simulink model "IEEE_39bus_genout"  (R2021a)
settings: Solver=ode3  StartTime=0.0  StopTime=100  FixedStep=Ts  MaxStep=1/60  RelTol=1e-2  AbsTol=1e-1
PreLoadFcn:
  | Ts=50e-6; ssn_ieee39_params; dec=20;
InitFcn:
  | Ts=50e-6; ssn_ieee39_params; dec=20;
values from neighbouring files (symbols this model uses):
  f = 50    [ssn_ieee39_params_ctrl.m]
  fNom = f    (= 60)    [ssn_ieee39_params_ctrl.m]
  ILR = 5.02    [ssn_ieee39_params_ctrl.m]
  IQMIN = 0.1    [ssn_ieee39_params_ctrl.m]
  ISCLIM = 1    [ssn_ieee39_params_ctrl.m]
  ITFpu = 1.10    (= 1.1)    [ssn_ieee39_params_ctrl.m]
  K = 1    [ssn_ieee39_params_ctrl.m]
  K1 = 1    [ssn_ieee39_params_ctrl.m]
  K2 = 2    [ssn_ieee39_params_ctrl.m]
  KCL = 1.04    [ssn_ieee39_params_ctrl.m]
  KFB = 0    [ssn_ieee39_params_ctrl.m]
  KFF = 1    [ssn_ieee39_params_ctrl.m]
  KFIX = 1    [ssn_ieee39_params_ctrl.m]
  KG = 1    [ssn_ieee39_params_ctrl.m]
  KIA = 59.91    [ssn_ieee39_params_ctrl.m]
  KIOEX = 0.0303    [ssn_ieee39_params_ctrl.m]
  KIUEX = 0.0303    [ssn_ieee39_params_ctrl.m]
  KIUOEX = 1    [ssn_ieee39_params_ctrl.m]
  KIUUEX = 1    [ssn_ieee39_params_ctrl.m]
  KLR = 22.47    [ssn_ieee39_params_ctrl.m]
  KM = 1    [ssn_ieee39_params_ctrl.m]
  KOEL = 0.24    [ssn_ieee39_params_ctrl.m]
  Kp = 1    [ssn_ieee39_params_ctrl.m]
  KPA = 30    [ssn_ieee39_params_ctrl.m]
  KPOEL = 1    [ssn_ieee39_params_ctrl.m]
  KPOEX = 0    [ssn_ieee39_params_ctrl.m]
  KPUEX = 0    [ssn_ieee39_params_ctrl.m]
  KSCALE = 0.319    [ssn_ieee39_params_ctrl.m]
  KUF = 0    [ssn_ieee39_params_ctrl.m]
  KUI = 0.001    [ssn_ieee39_params_ctrl.m]
  KUL = 0.24    [ssn_ieee39_params_ctrl.m]
  s = 10    [ssn_ieee39_params_ctrl.m]
  TA = 0.01    [ssn_ieee39_params_ctrl.m]
  Tadj = 0    [ssn_ieee39_params_ctrl.m]
  taps = [1 1 1.07 1.07 1.009 1.025 1 1.025 1.025 1.025]*1    [ssn_ieee39_params_ctrl.m]
  TF = 0.02    [ssn_ieee39_params_ctrl.m]
  TG = 0.024    [ssn_ieee39_params_ctrl.m]
  TINV = 0    [ssn_ieee39_params_ctrl.m]
  TIT = 0.1    [ssn_ieee39_params_ctrl.m]
  TL_10_11_len = 14    [ssn_ieee39_params_ctrl.m]
  TL_10_13_len = 14    [ssn_ieee39_params_ctrl.m]
  TL_13_14_len = 32    [ssn_ieee39_params_ctrl.m]
  TL_14_15_len = 70    [ssn_ieee39_params_ctrl.m]
  TL_15_16_len = 31.5    [ssn_ieee39_params_ctrl.m]
  TL_16_17_len = 26    [ssn_ieee39_params_ctrl.m]
  TL_16_19_len = 61    [ssn_ieee39_params_ctrl.m]
  TL_16_21_len = 46    [ssn_ieee39_params_ctrl.m]
  TL_16_24_len = 15    [ssn_ieee39_params_ctrl.m]
  TL_17_18_len = 26    [ssn_ieee39_params_ctrl.m]
  TL_17_27_len = 59    [ssn_ieee39_params_ctrl.m]
  TL_1_2_len = 134    [ssn_ieee39_params_ctrl.m]
  TL_1_39_len = 105    [ssn_ieee39_params_ctrl.m]
  TL_21_22_len = 47    [ssn_ieee39_params_ctrl.m]
  TL_22_23_len = 33    [ssn_ieee39_params_ctrl.m]
  TL_24_23_len = 88    [ssn_ieee39_params_ctrl.m]
  TL_25_26_len = 101    [ssn_ieee39_params_ctrl.m]
  TL_26_27_len = 46.5    [ssn_ieee39_params_ctrl.m]
  TL_26_28_len = 151    [ssn_ieee39_params_ctrl.m]
  TL_26_29_len = 200    [ssn_ieee39_params_ctrl.m]
  TL_28_29_len = 48    [ssn_ieee39_params_ctrl.m]
  TL_2_25_len = 28    [ssn_ieee39_params_ctrl.m]
  TL_2_2_len = 49    [ssn_ieee39_params_ctrl.m]
  TL_3_18_len = 42    [ssn_ieee39_params_ctrl.m]
  TL_3_4_len = 53    [ssn_ieee39_params_ctrl.m]
  TL_4_14_len = 33    [ssn_ieee39_params_ctrl.m]
  TL_4_5_len = 32.5    [ssn_ieee39_params_ctrl.m]
  TL_5_6_len = 14    [ssn_ieee39_params_ctrl.m]
  TL_5_8_len = 32    [ssn_ieee39_params_ctrl.m]
  TL_6_11_len = 26.5    [ssn_ieee39_params_ctrl.m]
  TL_6_7_len = 25.5    [ssn_ieee39_params_ctrl.m]
  TL_7_8_len = 15    [ssn_ieee39_params_ctrl.m]
  TL_8_9_len = 93    [ssn_ieee39_params_ctrl.m]
  TL_9_39_len = 136    [ssn_ieee39_params_ctrl.m]
  TOEL = 5.00    (= 5)    [ssn_ieee39_params_ctrl.m]
  TQREF = 0    [ssn_ieee39_params_ctrl.m]
  TQSCL = 0.012    [ssn_ieee39_params_ctrl.m]
  Ts_PMU = 1/1000    (= 0.001)    [ssn_ieee39_params_ctrl.m]
  TU1 = 0    [ssn_ieee39_params_ctrl.m]
  TU2 = 0    [ssn_ieee39_params_ctrl.m]
  TU3 = 0    [ssn_ieee39_params_ctrl.m]
  TU4 = 0    [ssn_ieee39_params_ctrl.m]
  TUL = 0    [ssn_ieee39_params_ctrl.m]
  TUP = 0.050    (= 0.05)    [ssn_ieee39_params_ctrl.m]
  TUQ = .005    (= 0.005)    [ssn_ieee39_params_ctrl.m]
  TUV = 0.2    [ssn_ieee39_params_ctrl.m]
  VAAMAX = VAMAX    (= 7.05)    [ssn_ieee39_params_ctrl.m]
  VAMAX = 7.05    [ssn_ieee39_params_ctrl.m]
  VAMIN = -6.11    [ssn_ieee39_params_ctrl.m]
  VBMAX = 999    [ssn_ieee39_params_ctrl.m]
  VF = 0    [ssn_ieee39_params_ctrl.m]
  VFB = 0    [ssn_ieee39_params_ctrl.m]
  VMMAX = 7.05    [ssn_ieee39_params_ctrl.m]
  VMMIN = -6.11    [ssn_ieee39_params_ctrl.m]
  VOELmax1 = 0.2353    [ssn_ieee39_params_ctrl.m]
  VOELmax2 = 0.0    (= 0)    [ssn_ieee39_params_ctrl.m]
  VOELmin1 = -0.24    [ssn_ieee39_params_ctrl.m]
  VOELmin2 = -1.0    (= -1)    [ssn_ieee39_params_ctrl.m]
  VRMAX = 7.05    [ssn_ieee39_params_ctrl.m]
  VRMIN = -6.11    [ssn_ieee39_params_ctrl.m]
  VSCLmax = 0.20    (= 0.2)    [ssn_ieee39_params_ctrl.m]
  VSCLmin = -0.10    (= -0.1)    [ssn_ieee39_params_ctrl.m]
  VUELmax1 = 1    [ssn_ieee39_params_ctrl.m]
  VUELmax2 = 1    [ssn_ieee39_params_ctrl.m]
  VUELmin1 = -1    [ssn_ieee39_params_ctrl.m]
  VUELmin2 = -1    [ssn_ieee39_params_ctrl.m]
  VUImax = 1    [ssn_ieee39_params_ctrl.m]
  VUImin = -1    [ssn_ieee39_params_ctrl.m]
undefined symbols (not defined in the file or in its folder): D1, Delta, MOV_segment9, powergui
libraries: spsThreePhaseVIMeasurementLib x42, slpidlib x40, powerlib_extras x30, op_dpl_lib x30, simulink_extras x20, spsST2AModel x20, spsThreePhaseParallelRLCLoadLib x19, spsThreePhaseTransformerTwoWindingsLib x13, spsSynchronousMachinepuStandardLib x10, simulink x10, spsPower3phInstantaneousLib x10, spsThreePhasePISectionLineLib x7
(part 5 of 12)

== system IEEE_39bus_genout/SM_master/G6/G6 ==
  note: Rotor Speed
  note: Rotor Speed Reference
  note: SM Measurement Signal
  note: Active Power
  note: Field Current
  note: Voltage Reference
  note: Stator Voltage
  note: Reactive Power
  note: Stator Current
  note: Field Voltage (Vf)
  note: Mechanical
      | Power (Pm)
  note: Measurement Outputs
  note: Rotor Speed
  note: Active Power
  note: Stator Voltage
  note: Stator Current
  note: Field Current
  note: Reactive Power
  wref (pu) : Inport
  Vref (pu) : Inport  Port=2
  Generator Measurements (Output) : Subsystem
  Governor model with Droop : Subsystem
  Ground7 : Ground
  ST6C EXCITER-1 : Subsystem
  Synchronous Machine : spsSynchronousMachinepuStandardLib/Synchronous Machine pu Standard  PresetModel=No  MechanicalLoad=Mechanical power Pm  ShowDetailedParameters=on  RotorType=Salient-pole  Units=per unit standard parameters  MeasurementBus=off  NominalParameters="[ Pn  Vn   f ]"  Reactances1=[ 31 32 33 34 35 36 37 ]  Reactances2=[ 1.305, 0.296, 0.252, 0.474, 0.243, 0.18 ]  dAxisTimeConstants=Short-circuit  qAxisTimeConstants=Open-circuit  TimeConstants1=[]  TimeConstants2=[]  TimeConstants3=[]  TimeConstants4=[]  TimeConstants5=[ 1.01, 0.053, 0.1 ]  TimeConstants6=[]  TimeConstants7=[]  TimeConstants8=[]  StatorResistance=2.8544e-3  Mechanical=[H1 0 2]  PolePairs=2  InitialConditions=[0 -62.5202 1.01055 1.01055 1.01055 8.25986 -111.74 128.26 1.32748]  SetSaturation=off  Saturation=[0.6404,0.7127,0.8441,0.9214,0.9956,1.082,1.19,1.316,1.457;0.7,0.7698,0.8872,0.9466,0.9969,1.046,1.1,1.151,1.201]  LoadFlowParameters=[1 150000000 0 0]  TsPowergui=0  TsBlock=-1  IterativeModel=Trapezoidal non iterative  IterativeDiscreteModel=Trapezoidal non iterative  BusType=PV  Pref=42e6  Qref=0  Qmin=-50000000  Qmax=50000000  PLF=0  QLF=0
      settings: SourceProductBaseCode=PS
  A : PMIOPort  Side=Right
  B : PMIOPort  Port=2  Side=Right
  C : PMIOPort  Port=3  Side=Right
  sm1 : Outport  VectorParamsAs1DForOutWhenUnconnected=off
  wires:
  [PT1st] -> Governor model with Droop/3(Input)
  [Ifd1st] -> ST6C EXCITER-1/4(Ifd)
  [Vt1st] -> ST6C EXCITER-1/2(Vt)
  [wm1] -> Governor model with Droop/2(w (pu))
  Generator Measurements (Output)/3(Vt) -> [Vt1st]
  Generator Measurements (Output)/6(PT) -> [PT1st]
  Generator Measurements (Output)/7(QT) -> [QT1st]
  Generator Measurements (Output)/1(sm) -> sm1/1
  Generator Measurements (Output)/5(It) -> [It1st]
  Generator Measurements (Output)/4(Ifd) -> [Ifd1st]
  Generator Measurements (Output)/2(wm) -> [wm1]
  ST6C EXCITER-1/1(Efd) -> Synchronous Machine/2, [Efd1st]
  [PT1st] -> ST6C EXCITER-1/7(PT)
  [It1st] -> ST6C EXCITER-1/3(It)
  [QT1st] -> ST6C EXCITER-1/6(QT)
  Ground7/1 -> ST6C EXCITER-1/5(Vstab)
  wref (pu)/1 -> Governor model with Droop/1(wref (pu)1)
  Governor model with Droop/1(Pmec (pu)) -> Synchronous Machine/1
  Vref (pu)/1 -> ST6C EXCITER-1/1(Vref)
  Synchronous Machine/1 -> Generator Measurements (Output)/1(m)
  connections:
  A/RConn1 -- Synchronous Machine/RConn1
  C/RConn1 -- Synchronous Machine/RConn3
  B/RConn1 -- Synchronous Machine/RConn2

== system IEEE_39bus_genout/SM_master/G7/G7 ==
  note: Rotor Speed
  note: Rotor Speed Reference
  note: SM Measurement Signal
  note: Active Power
  note: Field Current
  note: Voltage Reference
  note: Stator Voltage
  note: Reactive Power
  note: Stator Current
  note: Field Voltage (Vf)
  note: Mechanical
      | Power (Pm)
  note: Measurement Outputs
  note: Rotor Speed
  note: Active Power
  note: Stator Voltage
  note: Stator Current
  note: Field Current
  note: Reactive Power
  wref (pu) : Inport
  Vref (pu) : Inport  Port=2
  Generator Measurements (Output) : Subsystem
  Governor model with Droop : Subsystem
  Ground7 : Ground
  ST6C EXCITER-1 : Subsystem
  Synchronous Machine : spsSynchronousMachinepuStandardLib/Synchronous Machine pu Standard  PresetModel=No  MechanicalLoad=Mechanical power Pm  ShowDetailedParameters=on  RotorType=Salient-pole  Units=per unit standard parameters  MeasurementBus=off  NominalParameters="[ Pn  Vn   f ]"  Reactances1=[ 31 32 33 34 35 36 37 ]  Reactances2=[ 1.305, 0.296, 0.252, 0.474, 0.243, 0.18 ]  dAxisTimeConstants=Short-circuit  qAxisTimeConstants=Open-circuit  TimeConstants1=[]  TimeConstants2=[]  TimeConstants3=[]  TimeConstants4=[]  TimeConstants5=[ 1.01, 0.053, 0.1 ]  TimeConstants6=[]  TimeConstants7=[]  TimeConstants8=[]  StatorResistance=2.8544e-3  Mechanical=[H1 0 2]  PolePairs=2  InitialConditions=[0 -62.5202 1.01055 1.01055 1.01055 8.25986 -111.74 128.26 1.32748]  SetSaturation=off  Saturation=[0.6404,0.7127,0.8441,0.9214,0.9956,1.082,1.19,1.316,1.457;0.7,0.7698,0.8872,0.9466,0.9969,1.046,1.1,1.151,1.201]  LoadFlowParameters=[1 150000000 0 0]  TsPowergui=0  TsBlock=-1  IterativeModel=Trapezoidal non iterative  IterativeDiscreteModel=Trapezoidal non iterative  BusType=PV  Pref=42e6  Qref=0  Qmin=-50000000  Qmax=50000000  PLF=0  QLF=0
      settings: SourceProductBaseCode=PS
  A : PMIOPort  Side=Right
  B : PMIOPort  Port=2  Side=Right
  C : PMIOPort  Port=3  Side=Right
  sm1 : Outport  VectorParamsAs1DForOutWhenUnconnected=off
  wires:
  [PT1st] -> Governor model with Droop/3(Input)
  [Ifd1st] -> ST6C EXCITER-1/4(Ifd)
  [Vt1st] -> ST6C EXCITER-1/2(Vt)
  [wm1] -> Governor model with Droop/2(w (pu))
  Generator Measurements (Output)/3(Vt) -> [Vt1st]
  Generator Measurements (Output)/6(PT) -> [PT1st]
  Generator Measurements (Output)/7(QT) -> [QT1st]
  Generator Measurements (Output)/1(sm) -> sm1/1
  Generator Measurements (Output)/5(It) -> [It1st]
  Generator Measurements (Output)/4(Ifd) -> [Ifd1st]
  Generator Measurements (Output)/2(wm) -> [wm1]
  ST6C EXCITER-1/1(Efd) -> Synchronous Machine/2, [Efd1st]
  [PT1st] -> ST6C EXCITER-1/7(PT)
  [It1st] -> ST6C EXCITER-1/3(It)
  [QT1st] -> ST6C EXCITER-1/6(QT)
  Ground7/1 -> ST6C EXCITER-1/5(Vstab)
  wref (pu)/1 -> Governor model with Droop/1(wref (pu)1)
  Governor model with Droop/1(Pmec (pu)) -> Synchronous Machine/1
  Vref (pu)/1 -> ST6C EXCITER-1/1(Vref)
  Synchronous Machine/1 -> Generator Measurements (Output)/1(m)
  connections:
  A/RConn1 -- Synchronous Machine/RConn1
  C/RConn1 -- Synchronous Machine/RConn3
  B/RConn1 -- Synchronous Machine/RConn2

== system IEEE_39bus_genout/SM_master/G8/ G8 ==
  note: Reactive Power
  note: Field Current
  note: Stator Current
  note: Stator Voltage
  note: Active Power
  note: Rotor Speed
  note: Measurement Outputs
  note: Mechanical
      | Power (PU)
  note: Field Voltage (Vf PU)
  note: Stator Current
  note: Reactive Power
  note: Stator Voltage
  note: Voltage Reference
  note: Field Current
  note: Active Power
  note: SM Measurement Signal
  note: Rotor Speed Reference
  note: Rotor Speed
  wref (pu) : Inport
  Vref (pu) : Inport  Port=2
  "Generator Measurements " : Subsystem
  "Governor model " : Subsystem
  Ground7 : Ground
  ST6C EXCITER-1 : Subsystem
  Synchronous Machine : spsSynchronousMachinepuStandardLib/Synchronous Machine pu Standard  PresetModel=No  MechanicalLoad=Mechanical power Pm  ShowDetailedParameters=on  RotorType=Salient-pole  Units=per unit standard parameters  MeasurementBus=off  NominalParameters="[ Pn  Vn   f ]"  Reactances1=[ 31 32 33 34 35 36 37 ]  Reactances2=[ 1.305, 0.296, 0.252, 0.474, 0.243, 0.18 ]  dAxisTimeConstants=Short-circuit  qAxisTimeConstants=Open-circuit  TimeConstants1=[]  TimeConstants2=[]  TimeConstants3=[]  TimeConstants4=[]  TimeConstants5=[ 1.01, 0.053, 0.1 ]  TimeConstants6=[]  TimeConstants7=[]  TimeConstants8=[]  StatorResistance=2.8544e-3  Mechanical=[H1 0 2]  PolePairs=2  InitialConditions=[0 -62.5202 1.01055 1.01055 1.01055 8.25986 -111.74 128.26 1.32748]  SetSaturation=off  Saturation=[0.6404,0.7127,0.8441,0.9214,0.9956,1.082,1.19,1.316,1.457;0.7,0.7698,0.8872,0.9466,0.9969,1.046,1.1,1.151,1.201]  LoadFlowParameters=[1 150000000 0 0]  TsPowergui=0  TsBlock=-1  IterativeModel=Trapezoidal non iterative  IterativeDiscreteModel=Trapezoidal non iterative  BusType=PV  Pref=42e6  Qref=0  Qmin=-50000000  Qmax=50000000  PLF=0  QLF=0
      settings: SourceProductBaseCode=PS
  A : PMIOPort  Side=Right
  B : PMIOPort  Port=2  Side=Right
  C : PMIOPort  Port=3  Side=Right
  sm1 : Outport  VectorParamsAs1DForOutWhenUnconnected=off
  wires:
  Synchronous Machine/1 -> "Generator Measurements "/1(m)
  Vref (pu)/1 -> ST6C EXCITER-1/1(Vref)
  "Governor model "/1(Pmec (pu)) -> Synchronous Machine/1
  wref (pu)/1 -> "Governor model "/1(wref (pu)1)
  Ground7/1 -> ST6C EXCITER-1/5(Vstab)
  [QT1st] -> ST6C EXCITER-1/6(QT)
  [It1st] -> ST6C EXCITER-1/3(It)
  [PT1st] -> ST6C EXCITER-1/7(PT)
  ST6C EXCITER-1/1(Efd) -> [Efd1st], Synchronous Machine/2
  "Generator Measurements "/2(wm) -> [wm1]
  "Generator Measurements "/4(Ifd) -> [Ifd1st]
  "Generator Measurements "/5(It) -> [It1st]
  "Generator Measurements "/1(sm) -> sm1/1
  "Generator Measurements "/7(QT) -> [QT1st]
  "Generator Measurements "/6(PT) -> [PT1st]
  "Generator Measurements "/3(Vt) -> [Vt1st]
  [wm1] -> "Governor model "/2(w (pu))
  [Vt1st] -> ST6C EXCITER-1/2(Vt)
  [Ifd1st] -> ST6C EXCITER-1/4(Ifd)
  [PT1st] -> "Governor model "/3(Input)
  connections:
  B/RConn1 -- Synchronous Machine/RConn2
  C/RConn1 -- Synchronous Machine/RConn3
  A/RConn1 -- Synchronous Machine/RConn1

== system IEEE_39bus_genout/SM_master/G9/G9 ==
  note: Rotor Speed
  note: Rotor Speed Reference
  note: SM Measurement Signal
  note: Active Power
  note: Field Current
  note: Voltage Reference
  note: Stator Voltage
  note: Reactive Power
  note: Stator Current
  note: Field Voltage (Vf)
  note: Mechanical
      | Power (Pm)
  note: Measurement Outputs
  note: Rotor Speed
  note: Active Power
  note: Stator Voltage
  note: Stator Current
  note: Field Current
  note: Reactive Power
  wref (pu) : Inport
  Vref (pu) : Inport  Port=2
  Generator Measurements (Output) : Subsystem
  Governor model with Droop : Subsystem
  Ground7 : Ground
  ST6C EXCITER-1 : Subsystem
  Synchronous Machine : spsSynchronousMachinepuStandardLib/Synchronous Machine pu Standard  PresetModel=No  MechanicalLoad=Mechanical power Pm  ShowDetailedParameters=on  RotorType=Salient-pole  Units=per unit standard parameters  MeasurementBus=off  NominalParameters="[ Pn  Vn   f ]"  Reactances1=[ 31 32 33 34 35 36 37 ]  Reactances2=[ 1.305, 0.296, 0.252, 0.474, 0.243, 0.18 ]  dAxisTimeConstants=Short-circuit  qAxisTimeConstants=Open-circuit  TimeConstants1=[]  TimeConstants2=[]  TimeConstants3=[]  TimeConstants4=[]  TimeConstants5=[ 1.01, 0.053, 0.1 ]  TimeConstants6=[]  TimeConstants7=[]  TimeConstants8=[]  StatorResistance=2.8544e-3  Mechanical=[H1 0 2]  PolePairs=2  InitialConditions=[0 -62.5202 1.01055 1.01055 1.01055 8.25986 -111.74 128.26 1.32748]  SetSaturation=off  Saturation=[0.6404,0.7127,0.8441,0.9214,0.9956,1.082,1.19,1.316,1.457;0.7,0.7698,0.8872,0.9466,0.9969,1.046,1.1,1.151,1.201]  LoadFlowParameters=[1 150000000 0 0]  TsPowergui=0  TsBlock=-1  IterativeModel=Trapezoidal non iterative  IterativeDiscreteModel=Trapezoidal non iterative  BusType=PV  Pref=42e6  Qref=0  Qmin=-50000000  Qmax=50000000  PLF=0  QLF=0
      settings: SourceProductBaseCode=PS
  A : PMIOPort  Side=Right
  B : PMIOPort  Port=2  Side=Right
  C : PMIOPort  Port=3  Side=Right
  sm1 : Outport  VectorParamsAs1DForOutWhenUnconnected=off
  wires:
  [PT1st] -> Governor model with Droop/3(Input)
  [Ifd1st] -> ST6C EXCITER-1/4(Ifd)
  [Vt1st] -> ST6C EXCITER-1/2(Vt)
  [wm1] -> Governor model with Droop/2(w (pu))
  Generator Measurements (Output)/3(Vt) -> [Vt1st]
  Generator Measurements (Output)/6(PT) -> [PT1st]
  Generator Measurements (Output)/7(QT) -> [QT1st]
  Generator Measurements (Output)/1(sm) -> sm1/1
  Generator Measurements (Output)/5(It) -> [It1st]
  Generator Measurements (Output)/4(Ifd) -> [Ifd1st]
  Generator Measurements (Output)/2(wm) -> [wm1]
  ST6C EXCITER-1/1(Efd) -> Synchronous Machine/2, [Efd1st]
  [PT1st] -> ST6C EXCITER-1/7(PT)
  [It1st] -> ST6C EXCITER-1/3(It)
  [QT1st] -> ST6C EXCITER-1/6(QT)
  Ground7/1 -> ST6C EXCITER-1/5(Vstab)
  wref (pu)/1 -> Governor model with Droop/1(wref (pu)1)
  Governor model with Droop/1(Pmec (pu)) -> Synchronous Machine/1
  Vref (pu)/1 -> ST6C EXCITER-1/1(Vref)
  Synchronous Machine/1 -> Generator Measurements (Output)/1(m)
  connections:
  A/RConn1 -- Synchronous Machine/RConn1
  C/RConn1 -- Synchronous Machine/RConn3
  B/RConn1 -- Synchronous Machine/RConn2

== system IEEE_39bus_genout/powergui/EquivalentModel1/Sources ==
  Mux : Mux  Inputs=[1 1 1 1 1 1 1 1 1]
  u : Outport  VectorParamsAs1DForOutWhenUnconnected=off
  wires:
  Mux/1 -> u/1
  [T82_6949_9359448767590] -> Mux/1
  [T82_6950_9360569412504] -> Mux/2
  [T82_6951_9361932985223] -> Mux/3
  [T82_6951_9356282672159] -> Mux/4
  [T82_6952_9357399545649] -> Mux/5
  [T82_6953_9358759346944] -> Mux/6
  [T82_6951_9355573673919] -> Mux/7
  [T82_6952_9356690586475] -> Mux/8
  [T82_6953_9358050426837] -> Mux/9

== system IEEE_39bus_genout/powergui/EquivalentModel1/Yout ==
  v,i : Inport
  Demux : Demux  Outputs=[1 1 1 1 1 1 1 1 1 1 1 1]
  tag scope: T62_5432_5647820575465=global, T62_5433_5649868956552=global, T62_5434_5652472850936=global, T85_7307_11114326970370=global, T85_7308_11114868792739=global, T85_7309_11109720818426=global, T85_7309_11110395395566=global, T85_7309_11115651114168=global, T85_7310_11110259123535=global, T85_7310_11110933663860=global, T85_7311_11111037927703=global, T85_7311_11111712431213=global
  wires:
  v,i/1 -> Demux/1
  Demux/1 -> [T62_5432_5647820575465]
  Demux/2 -> [T62_5434_5652472850936]
  Demux/3 -> [T62_5433_5649868956552]
  Demux/4 -> [T85_7307_11114326970370]
  Demux/5 -> [T85_7308_11114868792739]
  Demux/6 -> [T85_7309_11115651114168]
  Demux/7 -> [T85_7309_11110395395566]
  Demux/8 -> [T85_7310_11110933663860]
  Demux/9 -> [T85_7311_11111712431213]
  Demux/10 -> [T85_7309_11109720818426]
  Demux/11 -> [T85_7310_11110259123535]
  Demux/12 -> [T85_7311_11111037927703]

== system IEEE_39bus_genout/powergui/EquivalentModel10/Sources ==
  Mux : Mux  Inputs=[1 1 1 1 1 1]
  u : Outport  VectorParamsAs1DForOutWhenUnconnected=off
  wires:
  Mux/1 -> u/1
  [T82_6950_9356943460879] -> Mux/1
  [T82_6951_9358062864679] -> Mux/2
  [T82_6952_9359425196284] -> Mux/3
  [T81_6898_9150624065361] -> Mux/4
  [T81_6899_9151655883262] -> Mux/5
  [T81_6900_9152927262892] -> Mux/6

== system IEEE_39bus_genout/powergui/EquivalentModel10/Yout ==
  v,i : Inport
  Demux : Demux  Outputs=[1 1 1 1 1 1 1 1 1]
  tag scope: T62_5433_5646980968421=global, T62_5434_5649027370724=global, T62_5435_5651629171655=global, T84_7256_10867012872856=global, T84_7257_10867470630205=global, T84_7258_10868165531364=global, T85_7308_11111622003241=global, T85_7309_11112162656022=global, T85_7310_11112943807863=global
  wires:
  v,i/1 -> Demux/1
  Demux/1 -> [T62_5433_5646980968421]
  Demux/2 -> [T62_5435_5651629171655]
  Demux/3 -> [T62_5434_5649027370724]
  Demux/4 -> [T85_7308_11111622003241]
  Demux/5 -> [T85_7309_11112162656022]
  Demux/6 -> [T85_7310_11112943807863]
  Demux/7 -> [T84_7256_10867012872856]
  Demux/8 -> [T84_7257_10867470630205]
  Demux/9 -> [T84_7258_10868165531364]

== system IEEE_39bus_genout/powergui/EquivalentModel11/Sources ==
  Mux : Mux  Inputs=[2 2 1 1 1]
  u : Outport  VectorParamsAs1DForOutWhenUnconnected=off
  wires:
  Mux/1 -> u/1
  [T71_6443_8452642742885] -> Mux/1
  [T71_6445_8448458918656] -> Mux/2
  [T82_6951_9356875498936] -> Mux/3
  [T82_6952_9357992177093] -> Mux/4
  [T82_6953_9359351783055] -> Mux/5

== system IEEE_39bus_genout/powergui/EquivalentModel11/Yout ==
  v,i : Inport
  Demux : Demux  Outputs=[2 2 1 1 1 1 1 1 1 1 1 1 1 1 1 1 1 1 1 1 1 1 1]
  tag scope: T61_5349_5543417394301=global, T61_5350_5545699742541=global, T61_5351_5548136384552=global, T61_5353_5538223301874=global, T61_5354_5540497361885=global, T61_5355_5542925715667=global, T62_5426_5654972758012=global, T62_5427_5653433505383=global, T62_5427_5657033058067=global, T62_5428_5655491826655=global, T62_5428_5659649562118=global, T62_5429_5658106237253=global, T62_5431_5647985538723=global, T62_5432_5650035991126=global, T62_5433_5652642076859=global, T62_5434_5646241082668=global, T62_5435_5648285506187=global, T62_5436_5650885213665=global, T71_6438_8383592831199=global, T71_6440_8379430192781=global, T85_7309_11110921551546=global, T85_7310_11111459635765=global, T85_7311_11112238219042=global
  wires:
  v,i/1 -> Demux/1
  Demux/1 -> [T71_6438_8383592831199]
  Demux/2 -> [T71_6440_8379430192781]
  Demux/3 -> [T62_5434_5646241082668]
  Demux/4 -> [T62_5436_5650885213665]
  Demux/5 -> [T62_5435_5648285506187]
  Demux/6 -> [T62_5426_5654972758012]
  Demux/7 -> [T62_5428_5659649562118]
  Demux/8 -> [T62_5427_5657033058067]
  Demux/9 -> [T62_5427_5653433505383]
  Demux/10 -> [T62_5429_5658106237253]
  Demux/11 -> [T62_5428_5655491826655]
  Demux/12 -> [T62_5431_5647985538723]
  Demux/13 -> [T62_5433_5652642076859]
  Demux/14 -> [T62_5432_5650035991126]
  Demux/15 -> [T85_7309_11110921551546]
  Demux/16 -> [T85_7310_11111459635765]
  Demux/17 -> [T85_7311_11112238219042]
  Demux/18 -> [T61_5349_5543417394301]
  Demux/19 -> [T61_5350_5545699742541]
  Demux/20 -> [T61_5351_5548136384552]
  Demux/21 -> [T61_5353_5538223301874]
  Demux/22 -> [T61_5354_5540497361885]
  Demux/23 -> [T61_5355_5542925715667]

== system IEEE_39bus_genout/powergui/EquivalentModel12/Sources ==
  Mux : Mux  Inputs=[1 1 1 1 1 1]
  u : Outport  VectorParamsAs1DForOutWhenUnconnected=off
  wires:
  Mux/1 -> u/1
  [T82_6944_9367677364306] -> Mux/1
  [T82_6945_9368807965179] -> Mux/2
  [T82_6946_9370181493857] -> Mux/3
  [T82_6940_9374445506138] -> Mux/4
  [T82_6941_9375583845193] -> Mux/5
  [T82_6942_9376965112052] -> Mux/6

== system IEEE_39bus_genout/powergui/EquivalentModel12/Yout ==
  v,i : Inport
  Demux : Demux  Outputs=[1 1 1 1 1 1 1 1 1]
  tag scope: T62_5429_5650654163998=global, T62_5430_5652708527702=global, T62_5431_5655318751393=global, T85_7298_11132912120499=global, T85_7299_11133470617289=global, T85_7300_11134269613137=global, T85_7302_11124581707193=global, T85_7303_11125132911756=global, T85_7304_11125924615378=global
  wires:
  v,i/1 -> Demux/1
  Demux/1 -> [T62_5429_5650654163998]
  Demux/2 -> [T62_5431_5655318751393]
  Demux/3 -> [T62_5430_5652708527702]
  Demux/4 -> [T85_7302_11124581707193]
  Demux/5 -> [T85_7303_11125132911756]
  Demux/6 -> [T85_7304_11125924615378]
  Demux/7 -> [T85_7298_11132912120499]
  Demux/8 -> [T85_7299_11133470617289]
  Demux/9 -> [T85_7300_11134269613137]

== system IEEE_39bus_genout/powergui/EquivalentModel13/Sources ==
  Mux : Mux  Inputs=[2 1 1 1 1 1 1]
  u : Outport  VectorParamsAs1DForOutWhenUnconnected=off
  wires:
  Mux/1 -> u/1
  [T71_6449_8440643700338] -> Mux/1
  [T82_6943_9369678820488] -> Mux/2
  [T82_6944_9370810857808] -> Mux/3
  [T82_6945_9372185822933] -> Mux/4
  [T82_6945_9365429130184] -> Mux/5
  [T82_6946_9366557591412] -> Mux/6
  [T82_6947_9367928980446] -> Mux/7

== system IEEE_39bus_genout/powergui/EquivalentModel13/Yout ==
  v,i : Inport
  Demux : Demux  Outputs=[2 1 1 1 1 1 1 1 1 1 1 1 1 1 1 1]
  tag scope: T61_5354_5537148912388=global, T61_5355_5539420888158=global, T61_5356_5541847157699=global, T62_5432_5646843574704=global, T62_5433_5645801331975=global, T62_5433_5648892048324=global, T62_5434_5647847826811=global, T62_5434_5651496040603=global, T62_5435_5650449725637=global, T71_6444_8371657346085=global, T85_7301_11126846508179=global, T85_7302_11127399066406=global, T85_7303_11121915074846=global, T85_7303_11128192123692=global, T85_7304_11122464263073=global, T85_7305_11123253950359=global
  wires:
  v,i/1 -> Demux/1
  Demux/1 -> [T71_6444_8371657346085]
  Demux/2 -> [T62_5432_5646843574704]
  Demux/3 -> [T62_5434_5651496040603]
  Demux/4 -> [T62_5433_5648892048324]
  Demux/5 -> [T62_5433_5645801331975]
  Demux/6 -> [T62_5435_5650449725637]
  Demux/7 -> [T62_5434_5647847826811]
  Demux/8 -> [T85_7301_11126846508179]
  Demux/9 -> [T85_7302_11127399066406]
  Demux/10 -> [T85_7303_11128192123692]
  Demux/11 -> [T85_7303_11121915074846]
  Demux/12 -> [T85_7304_11122464263073]
  Demux/13 -> [T85_7305_11123253950359]
  Demux/14 -> [T61_5354_5537148912388]
  Demux/15 -> [T61_5355_5539420888158]
  Demux/16 -> [T61_5356_5541847157699]

== system IEEE_39bus_genout/powergui/EquivalentModel14/Sources ==
  Mux : Mux  Inputs=[1 1 1 1 1 1]
  u : Outport  VectorParamsAs1DForOutWhenUnconnected=off
  wires:
  Mux/1 -> u/1
  [T82_6947_9362060579482] -> Mux/1
  [T82_6948_9363185230220] -> Mux/2
  [T82_6949_9364552808762] -> Mux/3
  [T82_6944_9366080142475] -> Mux/4
  [T82_6945_9367211134014] -> Mux/5
  [T82_6946_9368585053357] -> Mux/6

== system IEEE_39bus_genout/powergui/EquivalentModel14/Yout ==
  v,i : Inport
  Demux : Demux  Outputs=[1 1 1 1 1 1 1 1 1]
  tag scope: T62_5430_5649227224032=global, T62_5431_5651279655219=global, T62_5432_5653887834405=global, T85_7302_11123132587978=global, T85_7303_11123684160692=global, T85_7304_11124476232465=global, T85_7305_11117778837613=global, T85_7306_11118324434950=global, T85_7307_11119110531345=global
  wires:
  v,i/1 -> Demux/1
  Demux/1 -> [T62_5430_5649227224032]
  Demux/2 -> [T62_5432_5653887834405]
  Demux/3 -> [T62_5431_5651279655219]
  Demux/4 -> [T85_7305_11117778837613]
  Demux/5 -> [T85_7306_11118324434950]
  Demux/6 -> [T85_7307_11119110531345]
  Demux/7 -> [T85_7302_11123132587978]
  Demux/8 -> [T85_7303_11123684160692]
  Demux/9 -> [T85_7304_11124476232465]

== system IEEE_39bus_genout/powergui/EquivalentModel15/Sources ==
  Mux : Mux  Inputs=[2 1 1 1 1 1 1]
  u : Outport  VectorParamsAs1DForOutWhenUnconnected=off
  wires:
  Mux/1 -> u/1
  [T72_6483_8719846507879] -> Mux/1
  [T82_6948_9359112103368] -> Mux/2
  [T82_6949_9360235356725] -> Mux/3
  [T82_6950_9361601537888] -> Mux/4
  [T81_6894_9155974630444] -> Mux/5
  [T81_6895_9157014711401] -> Mux/6
  [T81_6896_9158294354086] -> Mux/7

== system IEEE_39bus_genout/powergui/EquivalentModel15/Yout ==
  v,i : Inport
  Demux : Demux  Outputs=[2 1 1 1 1 1 1 1 1 1 1 1 1 1 1 1]
  tag scope: T61_5356_5535304201612=global, T61_5357_5537572008902=global, T61_5358_5539994109962=global, T62_5431_5648273707774=global, T62_5432_5650324113911=global, T62_5433_5652930150695=global, T62_5434_5644858810537=global, T62_5435_5646903326589=global, T62_5436_5649503131962=global, T72_6478_8649276636039=global, T84_7252_10874089582357=global, T84_7253_10874555121014=global, T84_7254_10875257803481=global, T85_7306_11114610061787=global, T85_7307_11115154342275=global, T85_7308_11115939121821=global
  wires:
  v,i/1 -> Demux/1
  Demux/1 -> [T72_6478_8649276636039]
  Demux/2 -> [T62_5431_5648273707774]
  Demux/3 -> [T62_5433_5652930150695]
  Demux/4 -> [T62_5432_5650324113911]
  Demux/5 -> [T62_5434_5644858810537]
  Demux/6 -> [T62_5436_5649503131962]
  Demux/7 -> [T62_5435_5646903326589]
  Demux/8 -> [T85_7306_11114610061787]
  Demux/9 -> [T85_7307_11115154342275]
  Demux/10 -> [T85_7308_11115939121821]
  Demux/11 -> [T84_7252_10874089582357]
  Demux/12 -> [T84_7253_10874555121014]
  Demux/13 -> [T84_7254_10875257803481]
  Demux/14 -> [T61_5356_5535304201612]
  Demux/15 -> [T61_5357_5537572008902]
  Demux/16 -> [T61_5358_5539994109962]

== system IEEE_39bus_genout/powergui/EquivalentModel16/Sources ==
  Mux : Mux  Inputs=[1 1 1 1 1 1 1 1 1 1 1 1]
  u : Outport  VectorParamsAs1DForOutWhenUnconnected=off
  wires:
  Mux/1 -> u/1
  [T82_6949_9358454562471] -> Mux/1
  [T82_6950_9359575285518] -> Mux/2
  [T82_6951_9360938936370] -> Mux/3
  [T83_6995_9579324614907] -> Mux/4
  [T83_6996_9580544184534] -> Mux/5
  [T83_6997_9582010048378] -> Mux/6
  [T82_6951_9354413793574] -> Mux/7
  [T82_6952_9355531292129] -> Mux/8
  [T82_6953_9356891718488] -> Mux/9
  [T82_6952_9353179512093] -> Mux/10
  [T82_6953_9354295027269] -> Mux/11
  [T82_6954_9355653470250] -> Mux/12

== system IEEE_39bus_genout/powergui/EquivalentModel16/Yout ==
  v,i : Inport
  Demux : Demux  Outputs=[1 1 1 1 1 1 1 1 1 1 1 1 1 1 1 1 1 1 1 1 1]
  tag scope: T62_5432_5647233061597=global, T62_5433_5649281488950=global, T62_5434_5651885432282=global, T85_7307_11113386475406=global, T85_7308_11113928371406=global, T85_7309_11108738860471=global, T85_7309_11114710766465=global, T85_7310_11107086682655=global, T85_7310_11109277717807=global, T85_7311_11107623670916=global, T85_7311_11110057074202=global, T85_7312_11108401158235=global, T86_7353_11374789429948=global, T86_7354_11375424948722=global, T86_7355_11376304322380=global, T87_7749_11515247459914=global, T87_7750_11519185737637=global, T87_7751_11523365067314=global, T87_7761_11593912364935=global, T87_7762_11597817861518=global, T87_7763_11601964410056=global
  wires:
  v,i/1 -> Demux/1
  Demux/1 -> [T62_5432_5647233061597]
  Demux/2 -> [T62_5434_5651885432282]
  Demux/3 -> [T62_5433_5649281488950]
  Demux/4 -> [T85_7307_11113386475406]
  Demux/5 -> [T85_7308_11113928371406]
  Demux/6 -> [T85_7309_11114710766465]
  Demux/7 -> [T86_7353_11374789429948]
  Demux/8 -> [T86_7354_11375424948722]
  Demux/9 -> [T86_7355_11376304322380]
  Demux/10 -> [T85_7309_11108738860471]
  Demux/11 -> [T85_7310_11109277717807]
  Demux/12 -> [T85_7311_11110057074202]
  Demux/13 -> [T85_7310_11107086682655]
  Demux/14 -> [T85_7311_11107623670916]
  Demux/15 -> [T85_7312_11108401158235]
  Demux/16 -> [T87_7761_11593912364935]
  Demux/17 -> [T87_7762_11597817861518]
  Demux/18 -> [T87_7763_11601964410056]
  Demux/19 -> [T87_7749_11515247459914]
  Demux/20 -> [T87_7750_11519185737637]
  Demux/21 -> [T87_7751_11523365067314]

== system IEEE_39bus_genout/powergui/EquivalentModel17/Sources ==
  Mux : Mux  Inputs=[1 1 1 1 1 1]
  u : Outport  VectorParamsAs1DForOutWhenUnconnected=off
  wires:
  Mux/1 -> u/1
  [T82_6950_9356234429679] -> Mux/1
  [T82_6951_9357353872546] -> Mux/2
  [T82_6952_9358716243217] -> Mux/3
  [T83_6996_9578745878146] -> Mux/4
  [T83_6997_9579962907646] -> Mux/5
  [T83_6998_9581426231364] -> Mux/6

== system IEEE_39bus_genout/powergui/EquivalentModel17/Yout ==
  v,i : Inport
  Demux : Demux  Outputs=[1 1 1 1 1 1 1 1 1]
  tag scope: T62_5433_5646292136711=global, T62_5434_5648338585280=global, T62_5435_5650940435159=global, T85_7308_11110947395440=global, T85_7309_11111488085036=global, T85_7310_11112269273692=global, T86_7354_11373637319202=global, T86_7355_11374270442573=global, T86_7356_11375147420828=global
  wires:
  v,i/1 -> Demux/1
  Demux/1 -> [T62_5433_5646292136711]
  Demux/2 -> [T62_5435_5650940435159]
  Demux/3 -> [T62_5434_5648338585280]
  Demux/4 -> [T85_7308_11110947395440]
  Demux/5 -> [T85_7309_11111488085036]
  Demux/6 -> [T85_7310_11112269273692]
  Demux/7 -> [T86_7354_11373637319202]
  Demux/8 -> [T86_7355_11374270442573]
  Demux/9 -> [T86_7356_11375147420828]

== system IEEE_39bus_genout/powergui/EquivalentModel18/Sources ==
  Mux : Mux  Inputs=[1 1 1 1 1 1]
  u : Outport  VectorParamsAs1DForOutWhenUnconnected=off
  wires:
  Mux/1 -> u/1
  [T82_6952_9353751397422] -> Mux/1
  [T82_6953_9354866365667] -> Mux/2
  [T82_6954_9356224261716] -> Mux/3
  [T82_6954_9349609429678] -> Mux/4
  [T82_6955_9350721368762] -> Mux/5
  [T82_6956_9352076235652] -> Mux/6

== system IEEE_39bus_genout/powergui/EquivalentModel18/Yout ==
  v,i : Inport
  Demux : Demux  Outputs=[1 1 1 1 1 1 1 1 1]
  tag scope: T62_5434_5645450933115=global, T62_5435_5647495402901=global, T62_5436_5650095159326=global, T85_7310_11107510757479=global, T85_7311_11108047230328=global, T85_7312_11102811255989=global, T85_7312_11108824202235=global, T85_7313_11103344874249=global, T85_7314_11104118991569=global
  wires:
  v,i/1 -> Demux/1
  Demux/1 -> [T62_5434_5645450933115]
  Demux/2 -> [T62_5436_5650095159326]
  Demux/3 -> [T62_5435_5647495402901]
  Demux/4 -> [T85_7310_11107510757479]
  Demux/5 -> [T85_7311_11108047230328]
  Demux/6 -> [T85_7312_11108824202235]
  Demux/7 -> [T85_7312_11102811255989]
  Demux/8 -> [T85_7313_11103344874249]
  Demux/9 -> [T85_7314_11104118991569]

== system IEEE_39bus_genout/powergui/EquivalentModel19/Gates ==
  Mux : Mux  Inputs=[1 1 1]
  gates : Outport  VectorParamsAs1DForOutWhenUnconnected=off
  wires:
  Mux/1 -> gates/1
  [T60_5365_5468545752429] -> Mux/1
  [T60_5366_5471281698915] -> Mux/2
  [T60_5367_5474186626734] -> Mux/3

== system IEEE_39bus_genout/powergui/EquivalentModel19/Sources ==
  Mux : Mux  Inputs=[2 1 1 1 1 1 1]
  Mux_u : Mux  Inputs=[3 8]
  SwitchCurrents : Constant  Value=zeros(3,1)
  u : Outport  VectorParamsAs1DForOutWhenUnconnected=off
  wires:
  Mux_u/1 -> u/1
  SwitchCurrents/1 -> Mux_u/1
  Mux/1 -> Mux_u/2
  [T71_6453_8433565055541] -> Mux/1
  [T82_6953_9352515442590] -> Mux/2
  [T82_6954_9353628427456] -> Mux/3
  [T82_6955_9354984340126] -> Mux/4
  [T82_6955_9348942343071] -> Mux/5
  [T82_6956_9350051751846] -> Mux/6
  [T82_6957_9351404088425] -> Mux/7

== system IEEE_39bus_genout/powergui/EquivalentModel19/Status ==
  status : Inport
  Demux : Demux  Outputs=[1 1 1]
  tag scope: T62_5600_6294413145735=global, T62_5601_6296622043842=global, T62_5602_6298994472271=global
  wires:
  status/1 -> Demux/1
  Demux/1 -> [T62_5600_6294413145735]
  Demux/2 -> [T62_5601_6296622043842]
  Demux/3 -> [T62_5602_6298994472271]

== system IEEE_39bus_genout/powergui/EquivalentModel19/Yout ==
  v,i : Inport
  Demux : Demux  Outputs=[1 1 1 2 1 1 1 1 1 1 1 1 1 1 1 1 1 1 1]
  tag scope: T61_5357_5534533880322=global, T61_5358_5536799603372=global, T61_5359_5539219620191=global, T62_5435_5644016010389=global, T62_5435_5644709450809=global, T62_5436_5646058547657=global, T62_5436_5646751941811=global, T62_5437_5648656259577=global, T62_5437_5649349604783=global, T63_5699_6450445931111=global, T63_5700_6452462298341=global, T63_5701_6454639600174=global, T71_6448_8364621072909=global, T85_7311_11105857023025=global, T85_7312_11106391626798=global, T85_7313_11101578789692=global, T85_7313_11107166729630=global, T85_7314_11102110023465=global, T85_7315_11102881756297=global
  wires:
  v,i/1 -> Demux/1
  Demux/1 -> [T63_5699_6450445931111]
  Demux/2 -> [T63_5700_6452462298341]
  Demux/3 -> [T63_5701_6454639600174]
  Demux/4 -> [T71_6448_8364621072909]
  Demux/5 -> [T62_5435_5644709450809]
  Demux/6 -> [T62_5437_5649349604783]
  Demux/7 -> [T62_5436_5646751941811]
  Demux/8 -> [T62_5435_5644016010389]
  Demux/9 -> [T62_5437_5648656259577]
  Demux/10 -> [T62_5436_5646058547657]
  Demux/11 -> [T85_7311_11105857023025]
  Demux/12 -> [T85_7312_11106391626798]
  Demux/13 -> [T85_7313_11107166729630]
  Demux/14 -> [T85_7313_11101578789692]
  Demux/15 -> [T85_7314_11102110023465]
  Demux/16 -> [T85_7315_11102881756297]
  Demux/17 -> [T61_5357_5534533880322]
  Demux/18 -> [T61_5358_5536799603372]
  Demux/19 -> [T61_5359_5539219620191]

== system IEEE_39bus_genout/powergui/EquivalentModel2/Sources ==
  Mux : Mux  Inputs=[1 1 1 1 1 1]
  u : Outport  VectorParamsAs1DForOutWhenUnconnected=off
  wires:
  Mux/1 -> u/1
  [T80_6841_8955200428036] -> Mux/1
  [T80_6842_8956154264555] -> Mux/2
  [T80_6843_8957344297074] -> Mux/3
  [T81_6898_9150482046000] -> Mux/4
  [T81_6899_9151514101031] -> Mux/5
  [T81_6900_9152785717790] -> Mux/6

== system IEEE_39bus_genout/powergui/EquivalentModel2/Yout ==
  v,i : Inport
  Demux : Demux  Outputs=[1 1 1 1 1 1 1 1 1]
  tag scope: T61_5377_5536054307623=global, T61_5378_5537963739699=global, T61_5379_5540425032295=global, T83_7199_10635253179788=global, T83_7200_10635637190852=global, T83_7201_10636254991073=global, T84_7256_10866931061875=global, T84_7257_10867389042529=global, T84_7258_10868084166992=global
  wires:
  v,i/1 -> Demux/1
  Demux/1 -> [T61_5377_5536054307623]
  Demux/2 -> [T61_5379_5540425032295]
  Demux/3 -> [T61_5378_5537963739699]
  Demux/4 -> [T83_7199_10635253179788]
  Demux/5 -> [T83_7200_10635637190852]
  Demux/6 -> [T83_7201_10636254991073]
  Demux/7 -> [T84_7256_10866931061875]
  Demux/8 -> [T84_7257_10867389042529]
  Demux/9 -> [T84_7258_10868084166992]

== system IEEE_39bus_genout/powergui/EquivalentModel20/Sources ==
  Mux : Mux  Inputs=[1 1 1 1 1 1 1 1 1]
  u : Outport  VectorParamsAs1DForOutWhenUnconnected=off
  wires:
  Mux/1 -> u/1
  [T80_6843_8950965132239] -> Mux/1
  [T80_6844_8951915228403] -> Mux/2
  [T80_6845_8953101520568] -> Mux/3
  [T81_6897_9151353726086] -> Mux/4
  [T81_6898_9152388064250] -> Mux/5
  [T81_6899_9153661964142] -> Mux/6
  [T80_6844_8947711119328] -> Mux/7
  [T80_6845_8948659985112] -> Mux/8
  [T80_6846_8949845046897] -> Mux/9

== system IEEE_39bus_genout/powergui/EquivalentModel20/Yout ==
  v,i : Inport
  Demux : Demux  Outputs=[1 1 1 1 1 1 1 1 1 1 1 1 1 1 1]
  tag scope: T60_5301_5428489827898=global, T60_5302_5430616551624=global, T60_5303_5432894251684=global, T61_5379_5533137685492=global, T61_5380_5535043200847=global, T61_5381_5537500345279=global, T83_7201_10630306468722=global, T83_7202_10626886552154=global, T83_7202_10630686960068=global, T83_7203_10627265885698=global, T83_7203_10631301240570=global, T83_7204_10627879008398=global, T84_7255_10868301543368=global, T84_7256_10868761674045=global, T84_7257_10869458948531=global
  wires:
  v,i/1 -> Demux/1
  Demux/1 -> [T61_5379_5533137685492]
  Demux/2 -> [T61_5381_5537500345279]
  Demux/3 -> [T61_5380_5535043200847]
  Demux/4 -> [T83_7201_10630306468722]
  Demux/5 -> [T83_7202_10630686960068]
  Demux/6 -> [T83_7203_10631301240570]
  Demux/7 -> [T84_7255_10868301543368]
  Demux/8 -> [T84_7256_10868761674045]
  Demux/9 -> [T84_7257_10869458948531]
  Demux/10 -> [T83_7202_10626886552154]
  Demux/11 -> [T83_7203_10627265885698]
  Demux/12 -> [T83_7204_10627879008398]
  Demux/13 -> [T60_5301_5428489827898]
  Demux/14 -> [T60_5302_5430616551624]
  Demux/15 -> [T60_5303_5432894251684]

== system IEEE_39bus_genout/powergui/EquivalentModel21/Sources ==
  Mux : Mux  Inputs=[2 1 1 1 1 1 1 1 1 1 1 1 1]
  u : Outport  VectorParamsAs1DForOutWhenUnconnected=off
  wires:
  Mux/1 -> u/1
  [T71_6439_8461562821485] -> Mux/1
  [T80_6847_8943043044543] -> Mux/2
  [T80_6848_8943985659998] -> Mux/3
  [T80_6849_8945164471454] -> Mux/4
  [T80_6850_8937136957492] -> Mux/5
  [T80_6851_8938074442264] -> Mux/6
  [T80_6852_8939248123036] -> Mux/7
  [T81_6893_9157215730611] -> Mux/8
  [T81_6894_9158258529438] -> Mux/9
  [T81_6895_9159540889994] -> Mux/10
  [T80_6850_8936660163783] -> Mux/11
  [T80_6851_8937597808505] -> Mux/12
  [T80_6852_8938771649226] -> Mux/13

== system IEEE_39bus_genout/powergui/EquivalentModel21/Yout ==
  v,i : Inport
  Demux : Demux  Outputs=[2 1 1 1 1 1 1 1 1 1 1 1 1 1 1 1 1 1 1 1 1 1 1 1 1]
  tag scope: T61_5350_5542054606727=global, T61_5351_5544334919459=global, T61_5352_5546769525962=global, T61_5381_5530607750574=global, T61_5382_5529487790820=global, T61_5382_5532509349208=global, T61_5383_5531387431093=global, T61_5383_5534962345475=global, T61_5384_5533838353279=global, T62_5428_5652009758522=global, T62_5429_5654066147277=global, T62_5430_5656678513369=global, T71_6434_8392470538177=global, T83_7205_10620941972101=global, T83_7206_10621315424011=global, T83_7207_10621922665078=global, T83_7208_10613641942974=global, T83_7208_10614064271331=global, T83_7209_10614010717364=global, T83_7209_10614432895207=global, T83_7210_10614613280911=global, T83_7210_10615035308240=global, T84_7251_10875917366350=global, T84_7252_10876385464422=global, T84_7253_10877090706304=global
  wires:
  v,i/1 -> Demux/1
  Demux/1 -> [T71_6434_8392470538177]
  Demux/2 -> [T62_5428_5652009758522]
  Demux/3 -> [T62_5430_5656678513369]
  Demux/4 -> [T62_5429_5654066147277]
  Demux/5 -> [T61_5381_5530607750574]
  Demux/6 -> [T61_5383_5534962345475]
  Demux/7 -> [T61_5382_5532509349208]
  Demux/8 -> [T61_5382_5529487790820]
  Demux/9 -> [T61_5384_5533838353279]
  Demux/10 -> [T61_5383_5531387431093]
  Demux/11 -> [T83_7205_10620941972101]
  Demux/12 -> [T83_7206_10621315424011]
  Demux/13 -> [T83_7207_10621922665078]
  Demux/14 -> [T83_7208_10614064271331]
  Demux/15 -> [T83_7209_10614432895207]
  Demux/16 -> [T83_7210_10615035308240]
  Demux/17 -> [T84_7251_10875917366350]
  Demux/18 -> [T84_7252_10876385464422]
  Demux/19 -> [T84_7253_10877090706304]
  Demux/20 -> [T83_7208_10613641942974]
  Demux/21 -> [T83_7209_10614010717364]
  Demux/22 -> [T83_7210_10614613280911]
  Demux/23 -> [T61_5350_5542054606727]
  Demux/24 -> [T61_5351_5544334919459]
  Demux/25 -> [T61_5352_5546769525962]

== system IEEE_39bus_genout/powergui/EquivalentModel22/Sources ==
  Mux : Mux  Inputs=[2 1 1 1 1 1 1]
  u : Outport  VectorParamsAs1DForOutWhenUnconnected=off
  wires:
  Mux/1 -> u/1
  [T71_6437_8466299075855] -> Mux/1
  [T81_6899_9149750463735] -> Mux/2
  [T81_6900_9150779998503] -> Mux/3
  [T81_6901_9152049095000] -> Mux/4
  [T81_6906_9134485107778] -> Mux/5
  [T81_6907_9135503007994] -> Mux/6
  [T81_6908_9136760469938] -> Mux/7

== system IEEE_39bus_genout/powergui/EquivalentModel22/Yout ==
  v,i : Inport
  Demux : Demux  Outputs=[2 1 1 1 1 1 1 1 1 1 1 1 1 1 1 1]
  tag scope: T61_5352_5539591038760=global, T61_5353_5541867134279=global, T61_5354_5544297523568=global, T62_5430_5649414075241=global, T62_5431_5651466460161=global, T62_5432_5654074590399=global, T62_5436_5643272931531=global, T62_5437_5645313490016=global, T62_5438_5647909108482=global, T71_6432_8397185606736=global, T84_7257_10865640605422=global, T84_7258_10866096212748=global, T84_7259_10866788963884=global, T84_7264_10848225895747=global, T84_7265_10848670546832=global, T84_7266_10849352341725=global
  wires:
  v,i/1 -> Demux/1
  Demux/1 -> [T71_6432_8397185606736]
  Demux/2 -> [T62_5430_5649414075241]
  Demux/3 -> [T62_5432_5654074590399]
  Demux/4 -> [T62_5431_5651466460161]
  Demux/5 -> [T62_5436_5643272931531]
  Demux/6 -> [T62_5438_5647909108482]
  Demux/7 -> [T62_5437_5645313490016]
  Demux/8 -> [T84_7257_10865640605422]
  Demux/9 -> [T84_7258_10866096212748]
  Demux/10 -> [T84_7259_10866788963884]
  Demux/11 -> [T84_7264_10848225895747]
  Demux/12 -> [T84_7265_10848670546832]
  Demux/13 -> [T84_7266_10849352341725]
  Demux/14 -> [T61_5352_5539591038760]
  Demux/15 -> [T61_5353_5541867134279]
  Demux/16 -> [T61_5354_5544297523568]

== system IEEE_39bus_genout/powergui/EquivalentModel23/Sources ==
  Mux : Mux  Inputs=[1 1 1 1 1 1 1 1 1]
  u : Outport  VectorParamsAs1DForOutWhenUnconnected=off
  wires:
  Mux/1 -> u/1
  [T80_6845_8946912671074] -> Mux/1
  [T80_6846_8947859026884] -> Mux/2
  [T80_6847_8949041578695] -> Mux/3
  [T81_6894_9155446059111] -> Mux/4
  [T81_6895_9156486495762] -> Mux/5
  [T81_6896_9157766494142] -> Mux/6
  [T80_6846_8943844632847] -> Mux/7
  [T80_6847_8944789758277] -> Mux/8
  [T80_6848_8945971079707] -> Mux/9

== system IEEE_39bus_genout/powergui/EquivalentModel23/Yout ==
  v,i : Inport
  Demux : Demux  Outputs=[1 1 1 1 1 1 1 1 1 1 1 1 1 1 1]
  tag scope: T60_5302_5427239321907=global, T60_5303_5429363981006=global, T60_5304_5431639616438=global, T61_5380_5531824382131=global, T61_5381_5533727939126=global, T61_5382_5536183009475=global, T83_7203_10625536066159=global, T83_7204_10622295373923=global, T83_7204_10625913037787=global, T83_7205_10622671187749=global, T83_7205_10626523798572=global, T83_7206_10623280790732=global, T84_7252_10873662762765=global, T84_7253_10874128636380=global, T84_7254_10874831653804=global
  wires:
  v,i/1 -> Demux/1
  Demux/1 -> [T61_5380_5531824382131]
  Demux/2 -> [T61_5382_5536183009475]
  Demux/3 -> [T61_5381_5533727939126]
  Demux/4 -> [T83_7203_10625536066159]
  Demux/5 -> [T83_7204_10625913037787]
  Demux/6 -> [T83_7205_10626523798572]
  Demux/7 -> [T84_7252_10873662762765]
  Demux/8 -> [T84_7253_10874128636380]
  Demux/9 -> [T84_7254_10874831653804]
  Demux/10 -> [T83_7204_10622295373923]
  Demux/11 -> [T83_7205_10622671187749]
  Demux/12 -> [T83_7206_10623280790732]
  Demux/13 -> [T60_5302_5427239321907]
  Demux/14 -> [T60_5303_5429363981006]
  Demux/15 -> [T60_5304_5431639616438]

== system IEEE_39bus_genout/powergui/EquivalentModel24/Sources ==
  Mux : Mux  Inputs=[1 1 1 1 1 1 1 1 1]
  u : Outport  VectorParamsAs1DForOutWhenUnconnected=off
  wires:
  Mux/1 -> u/1
  [T80_6851_8936328954809] -> Mux/1
  [T80_6852_8937263929606] -> Mux/2
  [T80_6853_8938435100403] -> Mux/3
  [T80_6851_8935852295378] -> Mux/4
  [T80_6852_8936787430125] -> Mux/5
  [T80_6853_8937958760872] -> Mux/6
  [T80_6855_8929392884745] -> Mux/7
  [T80_6856_8930320538783] -> Mux/8
  [T80_6857_8931484388821] -> Mux/9

== system IEEE_39bus_genout/powergui/EquivalentModel24/Yout ==
  v,i : Inport
  Demux : Demux  Outputs=[1 1 1 1 1 1 1 1 1 1 1 1 1 1 1]
  tag scope: T61_5383_5528464502869=global, T61_5384_5527537886721=global, T61_5384_5530362184781=global, T61_5385_5529433610273=global, T61_5385_5532811032885=global, T61_5386_5531880384295=global, T83_7209_10612282709498=global, T83_7209_10612704913165=global, T83_7210_10612649121972=global, T83_7210_10613071175125=global, T83_7211_10613249323603=global, T83_7211_10613671226242=global, T83_7213_10604328680911=global, T83_7214_10604688053949=global, T83_7215_10605281216145=global
  wires:
  v,i/1 -> Demux/1
  Demux/1 -> [T61_5383_5528464502869]
  Demux/2 -> [T61_5385_5532811032885]
  Demux/3 -> [T61_5384_5530362184781]
  Demux/4 -> [T61_5384_5527537886721]
  Demux/5 -> [T61_5386_5531880384295]
  Demux/6 -> [T61_5385_5529433610273]
  Demux/7 -> [T83_7209_10612704913165]
  Demux/8 -> [T83_7210_10613071175125]
  Demux/9 -> [T83_7211_10613671226242]
  Demux/10 -> [T83_7209_10612282709498]
  Demux/11 -> [T83_7210_10612649121972]
  Demux/12 -> [T83_7211_10613249323603]
  Demux/13 -> [T83_7213_10604328680911]
  Demux/14 -> [T83_7214_10604688053949]
  Demux/15 -> [T83_7215_10605281216145]

== system IEEE_39bus_genout/powergui/EquivalentModel3/Sources ==
  Mux : Mux  Inputs=[2 1 1 1 1 1 1]
  u : Outport  VectorParamsAs1DForOutWhenUnconnected=off
  wires:
  Mux/1 -> u/1
  [T71_6447_8444459237807] -> Mux/1
  [T82_6941_9373800692853] -> Mux/2
  [T82_6942_9374936501597] -> Mux/3
  [T82_6943_9376315238147] -> Mux/4
  [T82_6942_9370326815676] -> Mux/5
  [T82_6943_9371461383306] -> Mux/6
  [T82_6944_9372838878741] -> Mux/7

== system IEEE_39bus_genout/powergui/EquivalentModel3/Yout ==
  v,i : Inport
  Demux : Demux  Outputs=[2 1 1 1 1 1 1 1 1 1 1 1 1 1 1 1]
  tag scope: T62_5400_5657033036700=global, T62_5401_5659464667702=global, T62_5402_5662053911930=global, T62_5428_5651993974045=global, T62_5429_5654050316534=global, T62_5430_5656662633678=global, T63_5478_5772208345228=global, T63_5479_5774413655550=global, T63_5480_5777178894424=global, T71_6442_8375451697742=global, T85_7299_11131700374006=global, T85_7300_11128061214644=global, T85_7300_11132256486308=global, T85_7301_11128616157359=global, T85_7301_11133053097669=global, T85_7302_11129411599132=global
  wires:
  v,i/1 -> Demux/1
  Demux/1 -> [T71_6442_8375451697742]
  Demux/2 -> [T62_5428_5651993974045]
  Demux/3 -> [T62_5430_5656662633678]
  Demux/4 -> [T62_5429_5654050316534]
  Demux/5 -> [T63_5478_5772208345228]
  Demux/6 -> [T63_5480_5777178894424]
  Demux/7 -> [T63_5479_5774413655550]
  Demux/8 -> [T85_7299_11131700374006]
  Demux/9 -> [T85_7300_11132256486308]
  Demux/10 -> [T85_7301_11133053097669]
  Demux/11 -> [T85_7300_11128061214644]
  Demux/12 -> [T85_7301_11128616157359]
  Demux/13 -> [T85_7302_11129411599132]
  Demux/14 -> [T62_5400_5657033036700]
  Demux/15 -> [T62_5401_5659464667702]
  Demux/16 -> [T62_5402_5662053911930]

== system IEEE_39bus_genout/powergui/EquivalentModel4/Sources ==
  Mux : Mux  Inputs=[2 1 1 1 1 1 1 1 1 1]
  u : Outport  VectorParamsAs1DForOutWhenUnconnected=off
  wires:
  Mux/1 -> u/1
  [T73_6533_8926023275864] -> Mux/1
  [T80_6840_8955992596188] -> Mux/2
  [T80_6841_8956948942682] -> Mux/3
  [T80_6842_8958141485176] -> Mux/4
  [T81_6895_9155249802994] -> Mux/5
  [T81_6896_9156287363688] -> Mux/6
  [T81_6897_9157564486111] -> Mux/7
  [T80_6842_8951760440441] -> Mux/8
  [T80_6843_8952713046581] -> Mux/9
  [T80_6844_8953901848720] -> Mux/10
